simulink model "First_App"  (R2023a)
settings: Solver=FixedStepDiscrete  StartTime=0.0  StopTime=inf  RelTol=1e-3
libraries: androiduilib x5, androidsensorlib x3, androidaudiovideolib x2
settings Model: Creator=parag  LastModifiedBy=parag
settings OptimizationCC: EnhancedBackFolding=on  PassReuseOutputArgsAs=Individual arguments  ZeroExternalMemoryAtStartup=off  ZeroInternalMemoryAtStartup=off  MaxStackSize=64  OptimizeBlockOrder=speed  DifferentSizesBufferReuse=on  OptimizationCustomize=off  EfficientTunableParamExpr=on
settings DebuggingCC: ParameterTunabilityLossMsg=error
settings HardwareCC: ProdBitPerPointer=32  ProdBitPerSizeT=32  ProdBitPerPtrDiffT=32  ProdLargestAtomicInteger=Long  ProdLargestAtomicFloat=Double  ProdWordSize=32  ProdHWDeviceType=ARM Compatible->ARM Cortex  UseEmbeddedCoderFeatures=off  UseSimulinkCoderFeatures=off
settings SFSimCC: MATLABDynamicMemAlloc=off
settings RTWCC: Description=Embedded Coder  SystemTargetFile=ert.tlc  HardwareBoard=Android Device  TLCOptions="-aInlineSetEventsForThisBaseRateFcn=TLC_FALSE -aSuppressMultiTaskScheduler=TLC_FALSE  -aRateBasedStepFcn=0"  TemplateMakefile=ert_default_tmf  RTWVerbose=off  Toolchain=Android SDK/NDK Tools
settings CodeAppCC: ForceParamTrailComments=on  IgnoreCustomStorageClasses=off  OperatorAnnotations=on  SimulinkDataObjDesc=on  SFDataObjDesc=on  InsertBlockDesc=on
settings ERTTargetCC: SupportNonInlinedSFcns=on

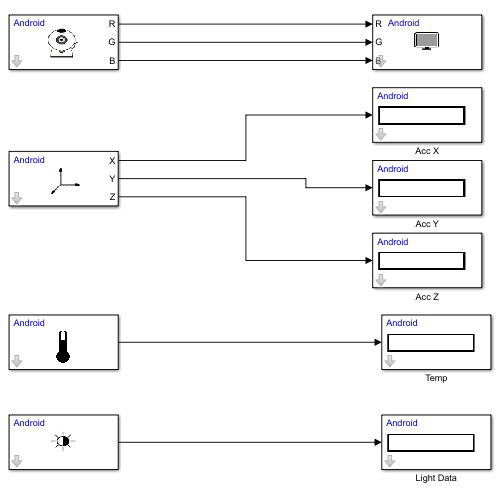
[thumbnail: Simulink's stored preview of the top-level diagram]
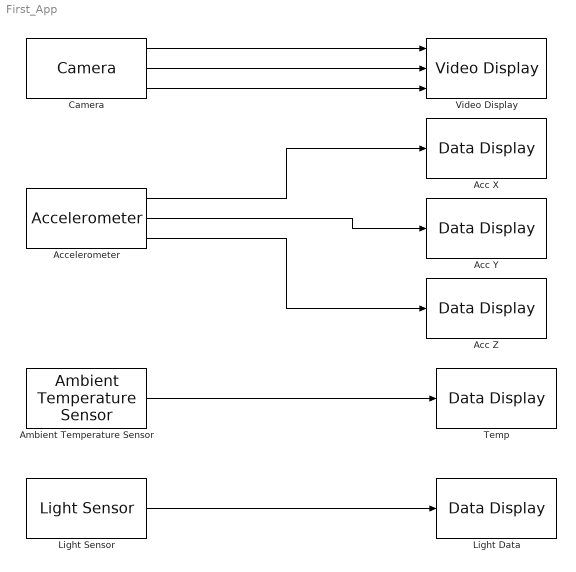
== system First_App ==
  Acc X : androiduilib/Data Display  DataDisplayId=First_App/Acc_X  Format=Float  Precision=6  SimulateUsing=Code generation  blockPlatform=Android
  Acc Y : androiduilib/Data Display  DataDisplayId=First_App/Acc_Y  Format=Float  Precision=6  SimulateUsing=Code generation  blockPlatform=Android
  Acc Z : androiduilib/Data Display  DataDisplayId=First_App/Acc_Z  Format=Float  Precision=6  SimulateUsing=Code generation  blockPlatform=Android
  Accelerometer : androidsensorlib/Accelerometer  OutputVector=off  SampleTime=0.1  BlockPlatform=Android
  Ambient Temperature Sensor : androidsensorlib/Ambient Temperature Sensor  SampleTime=0.1  BlockPlatform=Android
  Camera : androidaudiovideolib/Camera  CameraLocation=Back  CameraResolutions=Back - 1920x1080  Width=1920  Height=1080  SampleTime=0.001  BlockPlatform=Android
  Light Data : androiduilib/Data Display  DataDisplayId=First_App/Light_Data  Format=Float  Precision=6  SimulateUsing=Code generation  blockPlatform=Android
  Light Sensor : androidsensorlib/Light Sensor  SampleTime=0.1  BlockPlatform=Android
  Temp : androiduilib/Data Display  DataDisplayId=First_App/Temp  Format=Float  Precision=6  SimulateUsing=Code generation  blockPlatform=Android
  Video Display : androidaudiovideolib/Video Display  BlockPlatform=Android
  wires:
  Camera/1 -> Video Display/1
  Camera/2 -> Video Display/2
  Camera/3 -> Video Display/3
  Accelerometer/1 -> Acc X/1
  Accelerometer/2 -> Acc Y/1
  Accelerometer/3 -> Acc Z/1
  Ambient Temperature Sensor/1 -> Temp/1
  Light Sensor/1 -> Light Data/1
